simulink model "Model_Observador"  (R2022b)
settings: Solver=VariableStepAuto  StartTime=0.0  StopTime=10.0  RelTol=1e-3
values from neighbouring files (symbols this model uses):
  L = L'    [UAV.m]
undefined symbols (not defined in the file or in its folder): A, B, C, D, J
libraries: simulink x1
settings Model: Creator=samue  LastModifiedBy=samue

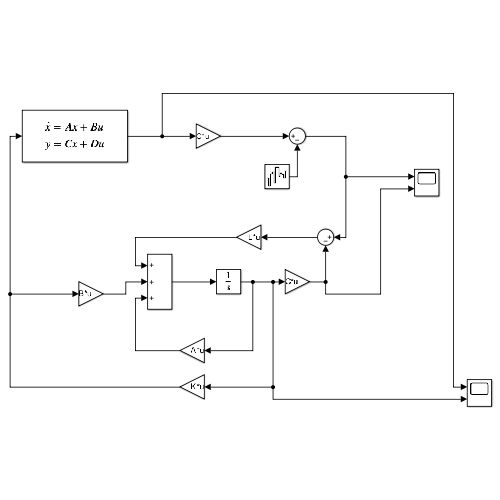
[thumbnail: Simulink's stored preview of the top-level diagram]
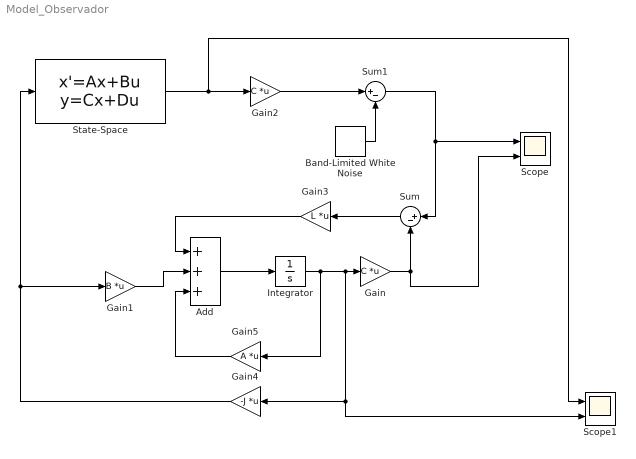
== system Model_Observador ==
  Add : Sum  Inputs=+++
  Band-Limited White Noise : simulink/Sources/Band-Limited White Noise  Cov=[1,1,1,1,1]*10e-6  Ts=0.01  seed=[23341]
  Gain : Gain  Gain=C  Multiplication=Matrix(K*u)
  Gain1 : Gain  Gain=B  Multiplication=Matrix(K*u)
  Gain2 : Gain  Gain=C  Multiplication=Matrix(K*u)
  Gain3 : Gain  Gain=L  Multiplication=Matrix(K*u)
  Gain4 : Gain  Gain=-J  Multiplication=Matrix(K*u)
  Gain5 : Gain  Gain=A  Multiplication=Matrix(K*u)
  Integrator : Integrator  InitialCondition=[-1, 0, 0, 0, 0]
  Scope : Scope  NumInputPorts=2
  Scope1 : Scope  NumInputPorts=2
  State-Space : StateSpace  A=A  B=B  C=C  D=D  InitialCondition=[-1, 0, 0, 0, 0]  ParameterTunability=Unconstrained
  Sum : Sum  Inputs=|+-
  Sum1 : Sum  Inputs=|+-
  wires:
  Gain2/1 -> Sum1/1
  Band-Limited White Noise/1 -> Sum1/2
  Sum1/1 -> Sum/1, Scope/1
  Sum/1 -> Gain3/1
  Gain/1 -> Scope/2, Sum/2
  Integrator/1 -> Gain5/1, Scope1/2, Gain4/1, Gain/1
  Add/1 -> Integrator/1
  Gain3/1 -> Add/1
  Gain1/1 -> Add/2
  Gain5/1 -> Add/3
  Gain4/1 -> Gain1/1, State-Space/1
  State-Space/1 -> Gain2/1, Scope1/1
